simulink model "n99tot98reg50neu"  (R2022b)
settings: Solver=VariableStepAuto  StartTime=0.0  StopTime=10.0  RelTol=1e-3
libraries: neural x56
(part 2 of 2)

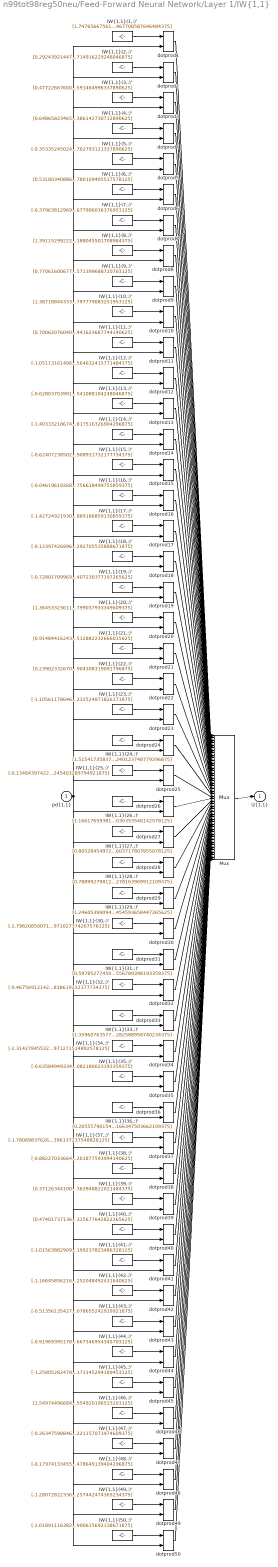
== system n99tot98reg50neu/Feed-Forward Neural Network/Layer 1/IW{1,1} ==
  "pd{1,1}" : Inport  PortDimensions=7
      mask Display: e = 0.06;c1 = [120 230 180]/255;c2 = ([120 230 180]+0)/(256+128);c3 = ([120 230 180]+128)/(256+128);patch([0 1 1 0],[0 0 1 1],c1);patch([0 1 1 1-e 1-e 0+e],[0 0 1 1-e 0+e 0+e],c2);patch([0 0 1 1-e 0+e 0+e],[0 1 1 1-e 1-e 0+e],c3);plot([0 1 1 0 0],[0 0 1 1 0]);
  "IW{1,1}(1,:)'" : Constant  Value=[1.747656675617606847339402520447038114070892333984375;0.49944644158864937022457297643995843827724456787109375;1.576232502923593070676133720553480088710784912109375;-0.265573401306849532499398947038571350276470184326171875;0.53099425991069237884545373162836767733097076416015625;-0.70547578790981491092537680742680095136165618896484375;-0.4153894187609112886860884827910922467708587646484375]
      mask Display: e = 0.06;c1 = [120 150 230]/255;c2 = ([120 150 230]+0)/383;c3 = ([120 150 230]+128)/383;patch([0 1 1 0],[0 0 1 1],c1);patch([0 1 1 1-e 1-e 0+e],[0 0 1 1-e 0+e 0+e],c2);patch([0 0 1 1-e 0+e 0+e],[0 1 1 1-e 1-e 0+e],c3);plot([0 1 1 0 0],[0 0 1 1 0]);disp('Weights');
  "IW{1,1}(10,:)'" : Constant  Value=[1.387188443330137577191862874315120279788970947265625;1.8579203813294060676497565509635023772716522216796875;-0.1472371632534580088158548960564075969159603118896484375;0.2709810301047463898527212222688831388950347900390625;-0.472918496976030555689618495307513512670993804931640625;0.277125353973486199254949724490870721638202667236328125;-0.5387110806703081511415120985475368797779083251953125]
      mask Display: e = 0.06;c1 = [120 150 230]/255;c2 = ([120 150 230]+0)/383;c3 = ([120 150 230]+128)/383;patch([0 1 1 0],[0 0 1 1],c1);patch([0 1 1 1-e 1-e 0+e],[0 0 1 1-e 0+e 0+e],c2);patch([0 0 1 1-e 0+e 0+e],[0 1 1 1-e 1-e 0+e],c3);plot([0 1 1 0 0],[0 0 1 1 0]);disp('Weights');
  "IW{1,1}(11,:)'" : Constant  Value=[0.7006207604086853724112415875424630939960479736328125;0.13393041436968455837330793656292371451854705810546875;2.002205300131398413299166350043378770351409912109375;3.592394854048140739877226224052719771862030029296875;-0.242048275446860861048747892709798179566860198974609375;-0.87313490454293984921463334103464148938655853271484375;0.79613684381734872719249551664688624441623687744140625]
      mask Display: e = 0.06;c1 = [120 150 230]/255;c2 = ([120 150 230]+0)/383;c3 = ([120 150 230]+128)/383;patch([0 1 1 0],[0 0 1 1],c1);patch([0 1 1 1-e 1-e 0+e],[0 0 1 1-e 0+e 0+e],c2);patch([0 0 1 1-e 0+e 0+e],[0 1 1 1-e 1-e 0+e],c3);plot([0 1 1 0 0],[0 0 1 1 0]);disp('Weights');
  "IW{1,1}(12,:)'" : Constant  Value=[-1.051131614068960828944909735582768917083740234375;-0.184968927308727160152557189576327800750732421875;-0.5549181350788590094680330366827547550201416015625;1.2416157312876137108759166949312202632427215576171875;-1.544207559212436020601444397470913827419281005859375;0.9759109470640339178970634748111478984355926513671875;-0.34009162520006286367646453072666190564632415771484375]
      mask Display: e = 0.06;c1 = [120 150 230]/255;c2 = ([120 150 230]+0)/383;c3 = ([120 150 230]+128)/383;patch([0 1 1 0],[0 0 1 1],c1);patch([0 1 1 1-e 1-e 0+e],[0 0 1 1-e 0+e 0+e],c2);patch([0 0 1 1-e 0+e 0+e],[0 1 1 1-e 1-e 0+e],c3);plot([0 1 1 0 0],[0 0 1 1 0]);disp('Weights');
  "IW{1,1}(13,:)'" : Constant  Value=[-0.62803703991998405253838200223981402814388275146484375;-1.8330351792178027903190695724333636462688446044921875;0.95103516127284659642526776224258355796337127685546875;-0.330923078802994929947800528680090792477130889892578125;-1.621712943876260748510276243905536830425262451171875;1.0999588154508710413637118108454160392284393310546875;0.379604016756278805910795881572994403541088104248046875]
      mask Display: e = 0.06;c1 = [120 150 230]/255;c2 = ([120 150 230]+0)/383;c3 = ([120 150 230]+128)/383;patch([0 1 1 0],[0 0 1 1],c1);patch([0 1 1 1-e 1-e 0+e],[0 0 1 1-e 0+e 0+e],c2);patch([0 0 1 1-e 0+e 0+e],[0 1 1 1-e 1-e 0+e],c3);plot([0 1 1 0 0],[0 0 1 1 0]);disp('Weights');
  "IW{1,1}(14,:)'" : Constant  Value=[-1.4033321867471306720887014307663775980472564697265625;0.28926622934015033816734785432345233857631683349609375;-0.05382639417858615937806376905427896417677402496337890625;-1.096686779105109366128090186975896358489990234375;-0.204014805347763228393631607104907743632793426513671875;0.045684822538907911282368701222367235459387302398681640625;-3.234885631069633671330620927619747817516326904296875]
      mask Display: e = 0.06;c1 = [120 150 230]/255;c2 = ([120 150 230]+0)/383;c3 = ([120 150 230]+128)/383;patch([0 1 1 0],[0 0 1 1],c1);patch([0 1 1 1-e 1-e 0+e],[0 0 1 1-e 0+e 0+e],c2);patch([0 0 1 1-e 0+e 0+e],[0 1 1 1-e 1-e 0+e],c3);plot([0 1 1 0 0],[0 0 1 1 0]);disp('Weights');
  "IW{1,1}(15,:)'" : Constant  Value=[-0.6240723850255258664532220791443251073360443115234375;0.077106870669531313300382180386804975569248199462890625;0.344852974648391763512478291886509396135807037353515625;-1.8315535668109468314668220045859925448894500732421875;1.7181195014105572482776551623828709125518798828125;1.23405048750804535728775590541772544384002685546875;1.243089227411525055089214220060966908931732177734375]
      mask Display: e = 0.06;c1 = [120 150 230]/255;c2 = ([120 150 230]+0)/383;c3 = ([120 150 230]+128)/383;patch([0 1 1 0],[0 0 1 1],c1);patch([0 1 1 1-e 1-e 0+e],[0 0 1 1-e 0+e 0+e],c2);patch([0 0 1 1-e 0+e 0+e],[0 1 1 1-e 1-e 0+e],c3);plot([0 1 1 0 0],[0 0 1 1 0]);disp('Weights');
  "IW{1,1}(16,:)'" : Constant  Value=[-0.0461961926841902015272722792360582388937473297119140625;-1.5178486125430044051398681403952650725841522216796875;0.88649917897524754817339953660848550498485565185546875;-1.694262860090099298560062379692681133747100830078125;-0.7956485499922798521055256060208193957805633544921875;-0.2040810857580830084412326641540857963263988494873046875;0.387239851931841128074296420891187153756618499755859375]
      mask Display: e = 0.06;c1 = [120 150 230]/255;c2 = ([120 150 230]+0)/383;c3 = ([120 150 230]+128)/383;patch([0 1 1 0],[0 0 1 1],c1);patch([0 1 1 1-e 1-e 0+e],[0 0 1 1-e 0+e 0+e],c2);patch([0 0 1 1-e 0+e 0+e],[0 1 1 1-e 1-e 0+e],c3);plot([0 1 1 0 0],[0 0 1 1 0]);disp('Weights');
  "IW{1,1}(17,:)'" : Constant  Value=[-1.427249219303456495566706507815979421138763427734375;0.55858969694210125478406325782998465001583099365234375;0.57312605493740698126003962897812016308307647705078125;1.6932739091869499770126594739849679172039031982421875;-0.00251143943317896738143257806541441823355853557586669921875;1.24398955198319516313176791300065815448760986328125;1.2629490962763778583166640601120889186859130859375]
      mask Display: e = 0.06;c1 = [120 150 230]/255;c2 = ([120 150 230]+0)/383;c3 = ([120 150 230]+128)/383;patch([0 1 1 0],[0 0 1 1],c1);patch([0 1 1 1-e 1-e 0+e],[0 0 1 1-e 0+e 0+e],c2);patch([0 0 1 1-e 0+e 0+e],[0 1 1 1-e 1-e 0+e],c3);plot([0 1 1 0 0],[0 0 1 1 0]);disp('Weights');
  "IW{1,1}(18,:)'" : Constant  Value=[-0.1239742699684905635759690767372376285493373870849609375;1.6475077386724310546384231201955117285251617431640625;-0.364087796388249118617608246495365165174007415771484375;1.1930065952474639967562097808695398271083831787109375;-0.7296279835965682192266967831528745591640472412109375;-1.9523779936641167953581543770269490778446197509765625;-2.11529792650099590645140779088251292705535888671875]
      mask Display: e = 0.06;c1 = [120 150 230]/255;c2 = ([120 150 230]+0)/383;c3 = ([120 150 230]+128)/383;patch([0 1 1 0],[0 0 1 1],c1);patch([0 1 1 1-e 1-e 0+e],[0 0 1 1-e 0+e 0+e],c2);patch([0 0 1 1-e 0+e 0+e],[0 1 1 1-e 1-e 0+e],c3);plot([0 1 1 0 0],[0 0 1 1 0]);disp('Weights');
  "IW{1,1}(19,:)'" : Constant  Value=[-0.72801709969798533705898080370388925075531005859375;-0.75685487829680064830739638637169264256954193115234375;-2.402055895370745819406010923557914793491363525390625;-4.40865217980332868563664305838756263256072998046875;1.788601743982917380293429232551716268062591552734375;-0.047649255890531087842543200849831919185817241668701171875;-0.54306338451648150655870495029375888407230377197265625]
      mask Display: e = 0.06;c1 = [120 150 230]/255;c2 = ([120 150 230]+0)/383;c3 = ([120 150 230]+128)/383;patch([0 1 1 0],[0 0 1 1],c1);patch([0 1 1 1-e 1-e 0+e],[0 0 1 1-e 0+e 0+e],c2);patch([0 0 1 1-e 0+e 0+e],[0 1 1 1-e 1-e 0+e],c3);plot([0 1 1 0 0],[0 0 1 1 0]);disp('Weights');
  "IW{1,1}(2,:)'" : Constant  Value=[0.2924392144750165289934784595970995724201202392578125;-1.487266421105410518777034667436964809894561767578125;1.227615355735253377389426532317884266376495361328125;0.477460046566002771495362821951857767999172210693359375;1.315340018711168124099231135915033519268035888671875;-0.493722517013425399312609442858956754207611083984375;-0.66240445347362164607574186447891406714916229248046875]
      mask Display: e = 0.06;c1 = [120 150 230]/255;c2 = ([120 150 230]+0)/383;c3 = ([120 150 230]+128)/383;patch([0 1 1 0],[0 0 1 1],c1);patch([0 1 1 1-e 1-e 0+e],[0 0 1 1-e 0+e 0+e],c2);patch([0 0 1 1-e 0+e 0+e],[0 1 1 1-e 1-e 0+e],c3);plot([0 1 1 0 0],[0 0 1 1 0]);disp('Weights');
  "IW{1,1}(20,:)'" : Constant  Value=[1.364533236116994618924991300445981323719024658203125;-1.0246759259485627158170473194331862032413482666015625;0.37029102084560083785191864080843515694141387939453125;-0.017143667388411464036490627904640859924256801605224609375;1.301862079554652940061032495577819645404815673828125;-0.73383683041816671899226776076829992234706878662109375;-0.307389929489428226361269480548799037933349609375]
      mask Display: e = 0.06;c1 = [120 150 230]/255;c2 = ([120 150 230]+0)/383;c3 = ([120 150 230]+128)/383;patch([0 1 1 0],[0 0 1 1],c1);patch([0 1 1 1-e 1-e 0+e],[0 0 1 1-e 0+e 0+e],c2);patch([0 0 1 1-e 0+e 0+e],[0 1 1 1-e 1-e 0+e],c3);plot([0 1 1 0 0],[0 0 1 1 0]);disp('Weights');
  "IW{1,1}(21,:)'" : Constant  Value=[0.9148441624371745906074693266418762505054473876953125;-2.26454895137788358994157533743418753147125244140625;0.92212391870621457368173423674306832253932952880859375;0.8388336282868242843591133350855670869350433349609375;-0.11914760626988642189250100500430562533438205718994140625;0.8434156135122823361172095246729440987110137939453125;1.3187282805795152995642638416029512882232666015625]
      mask Display: e = 0.06;c1 = [120 150 230]/255;c2 = ([120 150 230]+0)/383;c3 = ([120 150 230]+128)/383;patch([0 1 1 0],[0 0 1 1],c1);patch([0 1 1 1-e 1-e 0+e],[0 0 1 1-e 0+e 0+e],c2);patch([0 0 1 1-e 0+e 0+e],[0 1 1 1-e 1-e 0+e],c3);plot([0 1 1 0 0],[0 0 1 1 0]);disp('Weights');
  "IW{1,1}(22,:)'" : Constant  Value=[0.239023326709330297124012076892540790140628814697265625;1.63543700369563804741801504860632121562957763671875;-0.460467346974957225658187098815687932074069976806640625;-0.0152132308393917760336311317814761423505842685699462890625;1.8557407886556351872542336423066444694995880126953125;-0.145727466226683033401201328160823322832584381103515625;-1.4977839161156214498049621397512964904308319091796875]
      mask Display: e = 0.06;c1 = [120 150 230]/255;c2 = ([120 150 230]+0)/383;c3 = ([120 150 230]+128)/383;patch([0 1 1 0],[0 0 1 1],c1);patch([0 1 1 1-e 1-e 0+e],[0 0 1 1-e 0+e 0+e],c2);patch([0 0 1 1-e 0+e 0+e],[0 1 1 1-e 1-e 0+e],c3);plot([0 1 1 0 0],[0 0 1 1 0]);disp('Weights');
  "IW{1,1}(23,:)'" : Constant  Value=[-1.1056117864603602907180857073399238288402557373046875;-0.88512412117012928547410410828888416290283203125;-1.32691263005528536922383864293806254863739013671875;-0.353280134416258662088949904500623233616352081298828125;0.838270342845893967620440889731980860233306884765625;-1.1039078926360870180900519699207507073879241943359375;0.89537636960585487155839246042887680232524871826171875]
      mask Display: e = 0.06;c1 = [120 150 230]/255;c2 = ([120 150 230]+0)/383;c3 = ([120 150 230]+128)/383;patch([0 1 1 0],[0 0 1 1],c1);patch([0 1 1 1-e 1-e 0+e],[0 0 1 1-e 0+e 0+e],c2);patch([0 0 1 1-e 0+e 0+e],[0 1 1 1-e 1-e 0+e],c3);plot([0 1 1 0 0],[0 0 1 1 0]);disp('Weights');
  "IW{1,1}(24,:)'" : Constant  Value=[1.5154173583723322682459411225863732397556304931640625;1.24532548385659680434400797821581363677978515625;0.97493538415456082457666298068943433463573455810546875;-0.69399263410035072485726459490251727402210235595703125;0.28549801810493879994368171537644229829311370849609375;-0.07997892322433929057634571790913469158113002777099609375;0.64228307522436611787242100035655312240123748779296875]
      mask Display: e = 0.06;c1 = [120 150 230]/255;c2 = ([120 150 230]+0)/383;c3 = ([120 150 230]+128)/383;patch([0 1 1 0],[0 0 1 1],c1);patch([0 1 1 1-e 1-e 0+e],[0 0 1 1-e 0+e 0+e],c2);patch([0 0 1 1-e 0+e 0+e],[0 1 1 1-e 1-e 0+e],c3);plot([0 1 1 0 0],[0 0 1 1 0]);disp('Weights');
  "IW{1,1}(25,:)'" : Constant  Value=[-0.13484397422708671587798789914813823997974395751953125;-1.0885298201577475740720046815113164484500885009765625;-0.25682096877293603132130783706088550388813018798828125;0.039607047327919357726511151440718094818294048309326171875;0.11920677256356325413033658833228400908410549163818359375;-1.453256512868313254926988520310260355472564697265625;3.1420667487345621537997431005351245403289794921875]
      mask Display: e = 0.06;c1 = [120 150 230]/255;c2 = ([120 150 230]+0)/383;c3 = ([120 150 230]+128)/383;patch([0 1 1 0],[0 0 1 1],c1);patch([0 1 1 1-e 1-e 0+e],[0 0 1 1-e 0+e 0+e],c2);patch([0 0 1 1-e 0+e 0+e],[0 1 1 1-e 1-e 0+e],c3);plot([0 1 1 0 0],[0 0 1 1 0]);disp('Weights');
  "IW{1,1}(26,:)'" : Constant  Value=[1.166176593814495010548171194386668503284454345703125;1.4947985553874365560744763570255599915981292724609375;-0.54669401533347350419234089713427238166332244873046875;-2.468385339626232077847589607699774205684661865234375;0.2466663140045119162468978402102948166429996490478515625;-0.15218945163794017627623134103487245738506317138671875;-0.75219730552456021133167496373062022030353546142578125]
      mask Display: e = 0.06;c1 = [120 150 230]/255;c2 = ([120 150 230]+0)/383;c3 = ([120 150 230]+128)/383;patch([0 1 1 0],[0 0 1 1],c1);patch([0 1 1 1-e 1-e 0+e],[0 0 1 1-e 0+e 0+e],c2);patch([0 0 1 1-e 0+e 0+e],[0 1 1 1-e 1-e 0+e],c3);plot([0 1 1 0 0],[0 0 1 1 0]);disp('Weights');
  "IW{1,1}(27,:)'" : Constant  Value=[0.80528454972492713448417589461314491927623748779296875;0.58096862603202892305631621638895012438297271728515625;-1.5230858127770658949629023481975309550762176513671875;0.048101294679754651173464452540429192595183849334716796875;-1.9101916857836818142146739774034358561038970947265625;-0.294636196700321872921080057494691573083400726318359375;-1.00537860690854063960841813241131603717803955078125]
      mask Display: e = 0.06;c1 = [120 150 230]/255;c2 = ([120 150 230]+0)/383;c3 = ([120 150 230]+128)/383;patch([0 1 1 0],[0 0 1 1],c1);patch([0 1 1 1-e 1-e 0+e],[0 0 1 1-e 0+e 0+e],c2);patch([0 0 1 1-e 0+e 0+e],[0 1 1 1-e 1-e 0+e],c3);plot([0 1 1 0 0],[0 0 1 1 0]);disp('Weights');
  "IW{1,1}(28,:)'" : Constant  Value=[0.78899279812296618796807479156996123492717742919921875;-0.77936897219548451065662675318890251219272613525390625;1.6793369702174778534953247799421660602092742919921875;-0.360482007160921213984039468414266593754291534423828125;2.159602262172360287451056137797422707080841064453125;0.50602522395674631727757741828099824488162994384765625;0.74334678653509589363324039368308149278163909912109375]
      mask Display: e = 0.06;c1 = [120 150 230]/255;c2 = ([120 150 230]+0)/383;c3 = ([120 150 230]+128)/383;patch([0 1 1 0],[0 0 1 1],c1);patch([0 1 1 1-e 1-e 0+e],[0 0 1 1-e 0+e 0+e],c2);patch([0 0 1 1-e 0+e 0+e],[0 1 1 1-e 1-e 0+e],c3);plot([0 1 1 0 0],[0 0 1 1 0]);disp('Weights');
  "IW{1,1}(29,:)'" : Constant  Value=[1.246053990943079003983484653872437775135040283203125;-1.195940410100550632677141038584522902965545654296875;0.015527193852639557813954951370760682038962841033935546875;-0.01614452236154391429057142204328556545078754425048828125;1.8684337040291258968949250629520975053310394287109375;1.61290145209835866779712887364439666271209716796875;1.3569603838922239535946800970123149454593658447265625]
      mask Display: e = 0.06;c1 = [120 150 230]/255;c2 = ([120 150 230]+0)/383;c3 = ([120 150 230]+128)/383;patch([0 1 1 0],[0 0 1 1],c1);patch([0 1 1 1-e 1-e 0+e],[0 0 1 1-e 0+e 0+e],c2);patch([0 0 1 1-e 0+e 0+e],[0 1 1 1-e 1-e 0+e],c3);plot([0 1 1 0 0],[0 0 1 1 0]);disp('Weights');
  "IW{1,1}(3,:)'" : Constant  Value=[0.47722667600029800016869785395101644098758697509765625;-1.734739021348681742296093943878076970577239990234375;0.143811518424929174475579429781646467745304107666015625;1.5254287287772345660386008603381924331188201904296875;-1.094611060580545913722971818060614168643951416015625;0.400570644645104445569216977673931978642940521240234375;-0.64970032928261256532920242534601129591464996337890625]
      mask Display: e = 0.06;c1 = [120 150 230]/255;c2 = ([120 150 230]+0)/383;c3 = ([120 150 230]+128)/383;patch([0 1 1 0],[0 0 1 1],c1);patch([0 1 1 1-e 1-e 0+e],[0 0 1 1-e 0+e 0+e],c2);patch([0 0 1 1-e 0+e 0+e],[0 1 1 1-e 1-e 0+e],c3);plot([0 1 1 0 0],[0 0 1 1 0]);disp('Weights');
  "IW{1,1}(30,:)'" : Constant  Value=[-2.79820850071358773192287117126397788524627685546875;1.54179670863231788047187365009449422359466552734375;0.8064403497607031123806109462748281657695770263671875;0.351766777591807855429806295433081686496734619140625;-2.015346523677011614239518166868947446346282958984375;-1.2874435598761941879075720862601883709430694580078125;-1.4158899550481074403052161869709379971027374267578125]
      mask Display: e = 0.06;c1 = [120 150 230]/255;c2 = ([120 150 230]+0)/383;c3 = ([120 150 230]+128)/383;patch([0 1 1 0],[0 0 1 1],c1);patch([0 1 1 1-e 1-e 0+e],[0 0 1 1-e 0+e 0+e],c2);patch([0 0 1 1-e 0+e 0+e],[0 1 1 1-e 1-e 0+e],c3);plot([0 1 1 0 0],[0 0 1 1 0]);disp('Weights');
  "IW{1,1}(31,:)'" : Constant  Value=[0.59785277450840268453902126566390506923198699951171875;1.74409372320513256227059173397719860076904296875;0.354726683375673756959400861887843348085880279541015625;0.417731986711027125647177626888151280581951141357421875;-0.82909822929097909405271593641373328864574432373046875;-1.4865607481299563108478878348250873386859893798828125;-1.263156983701575253320470437756739556789398193359375]
      mask Display: e = 0.06;c1 = [120 150 230]/255;c2 = ([120 150 230]+0)/383;c3 = ([120 150 230]+128)/383;patch([0 1 1 0],[0 0 1 1],c1);patch([0 1 1 1-e 1-e 0+e],[0 0 1 1-e 0+e 0+e],c2);patch([0 0 1 1-e 0+e 0+e],[0 1 1 1-e 1-e 0+e],c3);plot([0 1 1 0 0],[0 0 1 1 0]);disp('Weights');
  "IW{1,1}(32,:)'" : Constant  Value=[-0.467569121426966216592546743413549847900867462158203125;1.071938363408374339513784434529952704906463623046875;1.1632653224053111085112277578446082770824432373046875;0.52729486405320835640253562814905308187007904052734375;1.0544362441029733190589467994868755340576171875;-0.33923970138657233430734549983753822743892669677734375;0.586796629949327464004227294935844838619232177734375]
      mask Display: e = 0.06;c1 = [120 150 230]/255;c2 = ([120 150 230]+0)/383;c3 = ([120 150 230]+128)/383;patch([0 1 1 0],[0 0 1 1],c1);patch([0 1 1 1-e 1-e 0+e],[0 0 1 1-e 0+e 0+e],c2);patch([0 0 1 1-e 0+e 0+e],[0 1 1 1-e 1-e 0+e],c3);plot([0 1 1 0 0],[0 0 1 1 0]);disp('Weights');
  "IW{1,1}(33,:)'" : Constant  Value=[1.3596076357733100081759403110481798648834228515625;-2.044468087476246864753193221986293792724609375;-1.1572914924628907584747139480896294116973876953125;-0.72656507570897621572925118016428314149379730224609375;0.42249878190688849866063492299872450530529022216796875;-1.0566425985453029579019812445039860904216766357421875;-0.82074728371824079431462450884282588958740234375]
      mask Display: e = 0.06;c1 = [120 150 230]/255;c2 = ([120 150 230]+0)/383;c3 = ([120 150 230]+128)/383;patch([0 1 1 0],[0 0 1 1],c1);patch([0 1 1 1-e 1-e 0+e],[0 0 1 1-e 0+e 0+e],c2);patch([0 0 1 1-e 0+e 0+e],[0 1 1 1-e 1-e 0+e],c3);plot([0 1 1 0 0],[0 0 1 1 0]);disp('Weights');
  "IW{1,1}(34,:)'" : Constant  Value=[-2.314278455329473072055179727612994611263275146484375;3.096416828243333529968595030368305742740631103515625;0.165424518369832906916627734972280450165271759033203125;-0.05617360352531756972904730673690210096538066864013671875;1.336202439871929659176430504885502159595489501953125;0.41390706623899287119883183549973182380199432373046875;-0.6797310280792523418114114974741823971271514892578125]
      mask Display: e = 0.06;c1 = [120 150 230]/255;c2 = ([120 150 230]+0)/383;c3 = ([120 150 230]+128)/383;patch([0 1 1 0],[0 0 1 1],c1);patch([0 1 1 1-e 1-e 0+e],[0 0 1 1-e 0+e 0+e],c2);patch([0 0 1 1-e 0+e 0+e],[0 1 1 1-e 1-e 0+e],c3);plot([0 1 1 0 0],[0 0 1 1 0]);disp('Weights');
  "IW{1,1}(35,:)'" : Constant  Value=[-0.6358494933411196203820736627676524221897125244140625;-1.5489992539573174124001297968789003789424896240234375;-1.70514848561234177992673721746541559696197509765625;-0.430721136624406308879287053059670142829418182373046875;-1.0048595441810526107673240403528325259685516357421875;-0.59747641019177766263936746327090077102184295654296875;0.43764038222769696684366635963669978082180023193359375]
      mask Display: e = 0.06;c1 = [120 150 230]/255;c2 = ([120 150 230]+0)/383;c3 = ([120 150 230]+128)/383;patch([0 1 1 0],[0 0 1 1],c1);patch([0 1 1 1-e 1-e 0+e],[0 0 1 1-e 0+e 0+e],c2);patch([0 0 1 1-e 0+e 0+e],[0 1 1 1-e 1-e 0+e],c3);plot([0 1 1 0 0],[0 0 1 1 0]);disp('Weights');
  "IW{1,1}(36,:)'" : Constant  Value=[0.205557901540687926189576728575048036873340606689453125;-1.223645094408394751184232518426142632961273193359375;0.95149708130478105605476457640179432928562164306640625;0.464250979591333601259606211897335015237331390380859375;1.3511428406536516444447215690161101520061492919921875;1.33131476326110220753662360948510468006134033203125;-1.6046192701498644961333184255636297166347503662109375]
      mask Display: e = 0.06;c1 = [120 150 230]/255;c2 = ([120 150 230]+0)/383;c3 = ([120 150 230]+128)/383;patch([0 1 1 0],[0 0 1 1],c1);patch([0 1 1 1-e 1-e 0+e],[0 0 1 1-e 0+e 0+e],c2);patch([0 0 1 1-e 0+e 0+e],[0 1 1 1-e 1-e 0+e],c3);plot([0 1 1 0 0],[0 0 1 1 0]);disp('Weights');
  "IW{1,1}(37,:)'" : Constant  Value=[-1.780898376261490057004266418516635894775390625;-0.618555182050433582929827025509439408779144287109375;-1.4373609083011322784528829288319684565067291259765625;0.90301859678045948154334610080695711076259613037109375;-0.07660094196647117270604354644092381931841373443603515625;-0.94962776800716774960875454780762083828449249267578125;0.87575113557798989205593898077495396137237548828125]
      mask Display: e = 0.06;c1 = [120 150 230]/255;c2 = ([120 150 230]+0)/383;c3 = ([120 150 230]+128)/383;patch([0 1 1 0],[0 0 1 1],c1);patch([0 1 1 1-e 1-e 0+e],[0 0 1 1-e 0+e 0+e],c2);patch([0 0 1 1-e 0+e 0+e],[0 1 1 1-e 1-e 0+e],c3);plot([0 1 1 0 0],[0 0 1 1 0]);disp('Weights');
  "IW{1,1}(38,:)'" : Constant  Value=[-0.882270336649107367321676065330393612384796142578125;0.04328286223777118302269428795625572092831134796142578125;-1.2646261397524563019345578140928409993648529052734375;0.922420917799984696472392897703684866428375244140625;-2.154867981227570172819696381338872015476226806640625;-0.966453858531078680016435100696980953216552734375;0.283468433100456496109842419173219241201877593994140625]
      mask Display: e = 0.06;c1 = [120 150 230]/255;c2 = ([120 150 230]+0)/383;c3 = ([120 150 230]+128)/383;patch([0 1 1 0],[0 0 1 1],c1);patch([0 1 1 1-e 1-e 0+e],[0 0 1 1-e 0+e 0+e],c2);patch([0 0 1 1-e 0+e 0+e],[0 1 1 1-e 1-e 0+e],c3);plot([0 1 1 0 0],[0 0 1 1 0]);disp('Weights');
  "IW{1,1}(39,:)'" : Constant  Value=[0.371263441006172756342351704006432555615901947021484375;0.53331155862665402533906444659805856645107269287109375;1.112038250172605824417360054212622344493865966796875;-0.73922509107107592374319438022212125360965728759765625;1.1841181266656504167400498772622086107730865478515625;0.9006643430544769568513174817780964076519012451171875;-1.591721705390868546459159915684722363948822021484375]
      mask Display: e = 0.06;c1 = [120 150 230]/255;c2 = ([120 150 230]+0)/383;c3 = ([120 150 230]+128)/383;patch([0 1 1 0],[0 0 1 1],c1);patch([0 1 1 1-e 1-e 0+e],[0 0 1 1-e 0+e 0+e],c2);patch([0 0 1 1-e 0+e 0+e],[0 1 1 1-e 1-e 0+e],c3);plot([0 1 1 0 0],[0 0 1 1 0]);disp('Weights');
  "IW{1,1}(4,:)'" : Constant  Value=[0.64865823465258376501196835306473076343536376953125;0.2344613740159174064547897842203383333981037139892578125;-0.48045487516191565102730010039522312581539154052734375;-1.2814031088295052551728758771787397563457489013671875;1.3399453094034914357735033263452351093292236328125;1.14153950468131082374156903824768960475921630859375;1.3336956324678974628028527149581350386142730712890625]
      mask Display: e = 0.06;c1 = [120 150 230]/255;c2 = ([120 150 230]+0)/383;c3 = ([120 150 230]+128)/383;patch([0 1 1 0],[0 0 1 1],c1);patch([0 1 1 1-e 1-e 0+e],[0 0 1 1-e 0+e 0+e],c2);patch([0 0 1 1-e 0+e 0+e],[0 1 1 1-e 1-e 0+e],c3);plot([0 1 1 0 0],[0 0 1 1 0]);disp('Weights');
  "IW{1,1}(40,:)'" : Constant  Value=[0.47401737136139654449351610310259275138378143310546875;0.1443753387717277292257023191268672235310077667236328125;-0.445205574153799521486263301994767971336841583251953125;1.4188919770855747959359405285795219242572784423828125;0.046202658139698045414167637545688194222748279571533203125;1.4128257188606887506665543696726672351360321044921875;-1.023024112720753553418262526975013315677642822265625]
      mask Display: e = 0.06;c1 = [120 150 230]/255;c2 = ([120 150 230]+0)/383;c3 = ([120 150 230]+128)/383;patch([0 1 1 0],[0 0 1 1],c1);patch([0 1 1 1-e 1-e 0+e],[0 0 1 1-e 0+e 0+e],c2);patch([0 0 1 1-e 0+e 0+e],[0 1 1 1-e 1-e 0+e],c3);plot([0 1 1 0 0],[0 0 1 1 0]);disp('Weights');
  "IW{1,1}(41,:)'" : Constant  Value=[-1.015638829099876350170461591915227472782135009765625;2.767053816463401982872483131359331309795379638671875;2.261356818364652188080299310968257486820220947265625;-0.1868634228738250413481836176288197748363018035888671875;0.719002057340242917149453205638565123081207275390625;-2.386032205980507026055192909552715718746185302734375;-5.22657363764995341881558488239534199237823486328125]
      mask Display: e = 0.06;c1 = [120 150 230]/255;c2 = ([120 150 230]+0)/383;c3 = ([120 150 230]+128)/383;patch([0 1 1 0],[0 0 1 1],c1);patch([0 1 1 1-e 1-e 0+e],[0 0 1 1-e 0+e 0+e],c2);patch([0 0 1 1-e 0+e 0+e],[0 1 1 1-e 1-e 0+e],c3);plot([0 1 1 0 0],[0 0 1 1 0]);disp('Weights');
  "IW{1,1}(42,:)'" : Constant  Value=[-1.16645856216911081304488106979988515377044677734375;-0.765914348274667755589462103671394288539886474609375;-1.147136650808885605101750115863978862762451171875;-0.4561023454182218106467416873783804476261138916015625;-1.131858827221291274867098763934336602687835693359375;-1.863473521467982951804742697277106344699859619140625;-0.48731753432313384966079183868714608252048492431640625]
      mask Display: e = 0.06;c1 = [120 150 230]/255;c2 = ([120 150 230]+0)/383;c3 = ([120 150 230]+128)/383;patch([0 1 1 0],[0 0 1 1],c1);patch([0 1 1 1-e 1-e 0+e],[0 0 1 1-e 0+e 0+e],c2);patch([0 0 1 1-e 0+e 0+e],[0 1 1 1-e 1-e 0+e],c3);plot([0 1 1 0 0],[0 0 1 1 0]);disp('Weights');
  "IW{1,1}(43,:)'" : Constant  Value=[-0.51356135427127591608353895935579203069210052490234375;-0.0380425272358840549369318750905222259461879730224609375;-1.1818972341017650595773602617555297911167144775390625;-1.6202277985747262079030406312085688114166259765625;-0.061381796748064897106811343974186456762254238128662109375;-0.12079960913816360779104996936439420096576213836669921875;1.2644207392429371861197751059080474078655242919921875]
      mask Display: e = 0.06;c1 = [120 150 230]/255;c2 = ([120 150 230]+0)/383;c3 = ([120 150 230]+128)/383;patch([0 1 1 0],[0 0 1 1],c1);patch([0 1 1 1-e 1-e 0+e],[0 0 1 1-e 0+e 0+e],c2);patch([0 0 1 1-e 0+e 0+e],[0 1 1 1-e 1-e 0+e],c3);plot([0 1 1 0 0],[0 0 1 1 0]);disp('Weights');
  "IW{1,1}(44,:)'" : Constant  Value=[-0.919693951786471064480110726435668766498565673828125;-0.63759504969468683288624788474407978355884552001953125;1.26303456644607781100830834475345909595489501953125;0.63964022040312962236185967412893660366535186767578125;0.77832391100262110494867329180124215781688690185546875;1.9202841680559898929203654915909282863140106201171875;-0.99090024817760646858033624084782786667346954345703125]
      mask Display: e = 0.06;c1 = [120 150 230]/255;c2 = ([120 150 230]+0)/383;c3 = ([120 150 230]+128)/383;patch([0 1 1 0],[0 0 1 1],c1);patch([0 1 1 1-e 1-e 0+e],[0 0 1 1-e 0+e 0+e],c2);patch([0 0 1 1-e 0+e 0+e],[0 1 1 1-e 1-e 0+e],c3);plot([0 1 1 0 0],[0 0 1 1 0]);disp('Weights');
  "IW{1,1}(45,:)'" : Constant  Value=[-1.25805282478053026551378934527747333049774169921875;0.87150745821274877567219618867966346442699432373046875;0.2542272804001601826939804595895111560821533203125;1.1438914335725669513266211652080528438091278076171875;1.5645877446592553194903985058772377669811248779296875;-0.55549203738715269285108888652757741510868072509765625;0.8576140225238664260842824660358019173145294189453125]
      mask Display: e = 0.06;c1 = [120 150 230]/255;c2 = ([120 150 230]+0)/383;c3 = ([120 150 230]+128)/383;patch([0 1 1 0],[0 0 1 1],c1);patch([0 1 1 1-e 1-e 0+e],[0 0 1 1-e 0+e 0+e],c2);patch([0 0 1 1-e 0+e 0+e],[0 1 1 1-e 1-e 0+e],c3);plot([0 1 1 0 0],[0 0 1 1 0]);disp('Weights');
  "IW{1,1}(46,:)'" : Constant  Value=[1.5497449668477685236211982555687427520751953125;-1.1408929307379047646264780269120819866657257080078125;0.35857627018847526567668637653696350753307342529296875;-2.64101483187210828162960751797072589397430419921875;1.223049071335231996471293314243666827678680419921875;1.37972539251158110573669546283781528472900390625;0.41703046322127346190455909891170449554920196533203125]
      mask Display: e = 0.06;c1 = [120 150 230]/255;c2 = ([120 150 230]+0)/383;c3 = ([120 150 230]+128)/383;patch([0 1 1 0],[0 0 1 1],c1);patch([0 1 1 1-e 1-e 0+e],[0 0 1 1-e 0+e 0+e],c2);patch([0 0 1 1-e 0+e 0+e],[0 1 1 1-e 1-e 0+e],c3);plot([0 1 1 0 0],[0 0 1 1 0]);disp('Weights');
  "IW{1,1}(47,:)'" : Constant  Value=[-0.263475988467886279575935759567073546350002288818359375;-0.86139482198021244396812790000694803893566131591796875;0.29975166291613042357511176305706612765789031982421875;1.426059500128983525968351386836729943752288818359375;0.9296813783801070041334924098919145762920379638671875;-0.46414727567939195740365221354295499622821807861328125;-0.45107432498225852324225115808076225221157073974609375]
      mask Display: e = 0.06;c1 = [120 150 230]/255;c2 = ([120 150 230]+0)/383;c3 = ([120 150 230]+128)/383;patch([0 1 1 0],[0 0 1 1],c1);patch([0 1 1 1-e 1-e 0+e],[0 0 1 1-e 0+e 0+e],c2);patch([0 0 1 1-e 0+e 0+e],[0 1 1 1-e 1-e 0+e],c3);plot([0 1 1 0 0],[0 0 1 1 0]);disp('Weights');
  "IW{1,1}(48,:)'" : Constant  Value=[-0.1797413345541949702965922597286407835781574249267578125;0.41897943081958433086953164092847146093845367431640625;-0.55505792894615446630979249675874598324298858642578125;-1.2853861057802060674504218695801682770252227783203125;-0.760985414848297292422785176313482224941253662109375;-0.951044710480042798650401891791261732578277587890625;-1.5098912287404064880291798544931225478649139404296875]
      mask Display: e = 0.06;c1 = [120 150 230]/255;c2 = ([120 150 230]+0)/383;c3 = ([120 150 230]+128)/383;patch([0 1 1 0],[0 0 1 1],c1);patch([0 1 1 1-e 1-e 0+e],[0 0 1 1-e 0+e 0+e],c2);patch([0 0 1 1-e 0+e 0+e],[0 1 1 1-e 1-e 0+e],c3);plot([0 1 1 0 0],[0 0 1 1 0]);disp('Weights');
  "IW{1,1}(49,:)'" : Constant  Value=[-1.2807282233641348323516240270691923797130584716796875;0.68915876955471688791732276513357646763324737548828125;0.2445756330386979759961008085156208835542201995849609375;1.2814935342341744473060316522605717182159423828125;0.406647322621566276179549959124415181577205657958984375;1.3771359623426366880494242650456726551055908203125;1.3778726877758324942391254808171652257442474365234375]
      mask Display: e = 0.06;c1 = [120 150 230]/255;c2 = ([120 150 230]+0)/383;c3 = ([120 150 230]+128)/383;patch([0 1 1 0],[0 0 1 1],c1);patch([0 1 1 1-e 1-e 0+e],[0 0 1 1-e 0+e 0+e],c2);patch([0 0 1 1-e 0+e 0+e],[0 1 1 1-e 1-e 0+e],c3);plot([0 1 1 0 0],[0 0 1 1 0]);disp('Weights');
  "IW{1,1}(5,:)'" : Constant  Value=[-0.353352450244067417539639563983655534684658050537109375;-0.433639085821924064045873592476709745824337005615234375;-0.90219050568865843953147987122065387666225433349609375;-0.2657325579975140517063891820725984871387481689453125;1.601768629363043761060225733672268688678741455078125;-1.3297896385042944356058569610468111932277679443359375;0.1862207972757463636526154004968702793121337890625]
      mask Display: e = 0.06;c1 = [120 150 230]/255;c2 = ([120 150 230]+0)/383;c3 = ([120 150 230]+128)/383;patch([0 1 1 0],[0 0 1 1],c1);patch([0 1 1 1-e 1-e 0+e],[0 0 1 1-e 0+e 0+e],c2);patch([0 0 1 1-e 0+e 0+e],[0 1 1 1-e 1-e 0+e],c3);plot([0 1 1 0 0],[0 0 1 1 0]);disp('Weights');
  "IW{1,1}(50,:)'" : Constant  Value=[-2.018911163828164490041672252118587493896484375;2.298443534595711046364385765627957880496978759765625;0.33520956691234216062724726725718937814235687255859375;1.2034240760566057293345920697902329266071319580078125;1.5925325800665455222571154081379063427448272705078125;-0.3031269859191016990962452837266027927398681640625;0.373687957622833522020044938471983186900615692138671875]
      mask Display: e = 0.06;c1 = [120 150 230]/255;c2 = ([120 150 230]+0)/383;c3 = ([120 150 230]+128)/383;patch([0 1 1 0],[0 0 1 1],c1);patch([0 1 1 1-e 1-e 0+e],[0 0 1 1-e 0+e 0+e],c2);patch([0 0 1 1-e 0+e 0+e],[0 1 1 1-e 1-e 0+e],c3);plot([0 1 1 0 0],[0 0 1 1 0]);disp('Weights');
  "IW{1,1}(6,:)'" : Constant  Value=[0.5318034088629299827033491965266875922679901123046875;-0.05717590530931339343201358360602171160280704498291015625;-0.94733840130549895608425003956654109060764312744140625;-0.0146788195354180840690450082774987095035612583160400390625;2.308522830923596114161000514286570250988006591796875;1.2037431893397132487422140911803580820560455322265625;-0.03790454788108706118965329778802697546780109405517578125]
      mask Display: e = 0.06;c1 = [120 150 230]/255;c2 = ([120 150 230]+0)/383;c3 = ([120 150 230]+128)/383;patch([0 1 1 0],[0 0 1 1],c1);patch([0 1 1 1-e 1-e 0+e],[0 0 1 1-e 0+e 0+e],c2);patch([0 0 1 1-e 0+e 0+e],[0 1 1 1-e 1-e 0+e],c3);plot([0 1 1 0 0],[0 0 1 1 0]);disp('Weights');
  "IW{1,1}(7,:)'" : Constant  Value=[-0.379638129699689186313804611927480436861515045166015625;0.5398169246130877230172018244047649204730987548828125;1.140584439302090746792828213074244558811187744140625;0.61722127131611637107511114663793705403804779052734375;1.3606223929806964267896773890242911875247955322265625;0.56343294578792069149386634308029897511005401611328125;0.97896543814351677514906668875482864677906036376953125]
      mask Display: e = 0.06;c1 = [120 150 230]/255;c2 = ([120 150 230]+0)/383;c3 = ([120 150 230]+128)/383;patch([0 1 1 0],[0 0 1 1],c1);patch([0 1 1 1-e 1-e 0+e],[0 0 1 1-e 0+e 0+e],c2);patch([0 0 1 1-e 0+e 0+e],[0 1 1 1-e 1-e 0+e],c3);plot([0 1 1 0 0],[0 0 1 1 0]);disp('Weights');
  "IW{1,1}(8,:)'" : Constant  Value=[1.3911529922247594104334211806417442858219146728515625;-3.108901065696418442030335427261888980865478515625;-2.56068493120445506150417713797651231288909912109375;-0.476377804219743572478051873986260034143924713134765625;0.5930594051890292206508092931471765041351318359375;-1.5123935503399625890352808710304088890552520751953125;0.958351638789282755936937974183820188045501708984375]
      mask Display: e = 0.06;c1 = [120 150 230]/255;c2 = ([120 150 230]+0)/383;c3 = ([120 150 230]+128)/383;patch([0 1 1 0],[0 0 1 1],c1);patch([0 1 1 1-e 1-e 0+e],[0 0 1 1-e 0+e 0+e],c2);patch([0 0 1 1-e 0+e 0+e],[0 1 1 1-e 1-e 0+e],c3);plot([0 1 1 0 0],[0 0 1 1 0]);disp('Weights');
  "IW{1,1}(9,:)'" : Constant  Value=[0.770616006774930806244583436637185513973236083984375;-1.3223955779284024547592935050488449633121490478515625;-1.6183259513531871309766074773506261408329010009765625;1.5763537694544391687401230228715576231479644775390625;-1.1200073332976734352683934048400260508060455322265625;1.4510169135761297187769969241344369947910308837890625;0.7298236116551006791297595555079169571399688720703125]
      mask Display: e = 0.06;c1 = [120 150 230]/255;c2 = ([120 150 230]+0)/383;c3 = ([120 150 230]+128)/383;patch([0 1 1 0],[0 0 1 1],c1);patch([0 1 1 1-e 1-e 0+e],[0 0 1 1-e 0+e 0+e],c2);patch([0 0 1 1-e 0+e 0+e],[0 1 1 1-e 1-e 0+e],c3);plot([0 1 1 0 0],[0 0 1 1 0]);disp('Weights');
  Mux : Mux  Inputs=50
      mask Display: e = 0.06;c1 = [120 150 230]/255;c2 = ([120 150 230]+0)/383;c3 = ([120 150 230]+128)/383;patch([0 1 1 0],[0 0 1 1],c1);patch([0 1 1 1-e 1-e 0+e],[0 0 1 1-e 0+e 0+e],c2);patch([0 0 1 1-e 0+e 0+e],[0 1 1 1-e 1-e 0+e],c3);plot([0 1 1 0 0],[0 0 1 1 0]);disp('Mux');
  dotprod{1..50} (50 alike) : neural/Weight Functions/dotprod
  "iz{1,1}" : Outport
      mask Display: e = 0.06;c1 = [120 230 180]/255;c2 = ([120 230 180]+0)/(256+128);c3 = ([120 230 180]+128)/(256+128);patch([0 1 1 0],[0 0 1 1],c1);patch([0 1 1 1-e 1-e 0+e],[0 0 1 1-e 0+e 0+e],c2);patch([0 0 1 1-e 0+e 0+e],[0 1 1 1-e 1-e 0+e],c3);plot([0 1 1 0 0],[0 0 1 1 0]);
  wires:
  "IW{1,1}(1,:)'"/1 -> dotprod1/1
  "pd{1,1}"/1 -> dotprod1/2, dotprod2/2, dotprod3/2, dotprod4/2, dotprod5/2, dotprod6/2, dotprod7/2, dotprod8/2, dotprod9/2, dotprod10/2, dotprod11/2, dotprod12/2, dotprod13/2, dotprod14/2, dotprod15/2, dotprod16/2, dotprod17/2, dotprod18/2, dotprod19/2, dotprod20/2, dotprod21/2, dotprod22/2, dotprod23/2, dotprod24/2, dotprod25/2, dotprod26/2, dotprod27/2, dotprod28/2, dotprod29/2, dotprod30/2, dotprod31/2, dotprod32/2, dotprod33/2, dotprod34/2, dotprod35/2, dotprod36/2, dotprod37/2, dotprod38/2, dotprod39/2, dotprod40/2, dotprod41/2, dotprod42/2, dotprod43/2, dotprod44/2, dotprod45/2, dotprod46/2, dotprod47/2, dotprod48/2, dotprod49/2, dotprod50/2
  dotprod1/1 -> Mux/1
  "IW{1,1}(2,:)'"/1 -> dotprod2/1
  dotprod2/1 -> Mux/2
  "IW{1,1}(3,:)'"/1 -> dotprod3/1
  dotprod3/1 -> Mux/3
  "IW{1,1}(4,:)'"/1 -> dotprod4/1
  dotprod4/1 -> Mux/4
  "IW{1,1}(5,:)'"/1 -> dotprod5/1
  dotprod5/1 -> Mux/5
  "IW{1,1}(6,:)'"/1 -> dotprod6/1
  dotprod6/1 -> Mux/6
  "IW{1,1}(7,:)'"/1 -> dotprod7/1
  dotprod7/1 -> Mux/7
  "IW{1,1}(8,:)'"/1 -> dotprod8/1
  dotprod8/1 -> Mux/8
  "IW{1,1}(9,:)'"/1 -> dotprod9/1
  dotprod9/1 -> Mux/9
  "IW{1,1}(10,:)'"/1 -> dotprod10/1
  dotprod10/1 -> Mux/10
  "IW{1,1}(11,:)'"/1 -> dotprod11/1
  dotprod11/1 -> Mux/11
  "IW{1,1}(12,:)'"/1 -> dotprod12/1
  dotprod12/1 -> Mux/12
  "IW{1,1}(13,:)'"/1 -> dotprod13/1
  dotprod13/1 -> Mux/13
  "IW{1,1}(14,:)'"/1 -> dotprod14/1
  dotprod14/1 -> Mux/14
  "IW{1,1}(15,:)'"/1 -> dotprod15/1
  dotprod15/1 -> Mux/15
  "IW{1,1}(16,:)'"/1 -> dotprod16/1
  dotprod16/1 -> Mux/16
  "IW{1,1}(17,:)'"/1 -> dotprod17/1
  dotprod17/1 -> Mux/17
  "IW{1,1}(18,:)'"/1 -> dotprod18/1
  dotprod18/1 -> Mux/18
  "IW{1,1}(19,:)'"/1 -> dotprod19/1
  dotprod19/1 -> Mux/19
  "IW{1,1}(20,:)'"/1 -> dotprod20/1
  dotprod20/1 -> Mux/20
  "IW{1,1}(21,:)'"/1 -> dotprod21/1
  dotprod21/1 -> Mux/21
  "IW{1,1}(22,:)'"/1 -> dotprod22/1
  dotprod22/1 -> Mux/22
  "IW{1,1}(23,:)'"/1 -> dotprod23/1
  dotprod23/1 -> Mux/23
  "IW{1,1}(24,:)'"/1 -> dotprod24/1
  dotprod24/1 -> Mux/24
  "IW{1,1}(25,:)'"/1 -> dotprod25/1
  dotprod25/1 -> Mux/25
  "IW{1,1}(26,:)'"/1 -> dotprod26/1
  dotprod26/1 -> Mux/26
  "IW{1,1}(27,:)'"/1 -> dotprod27/1
  dotprod27/1 -> Mux/27
  "IW{1,1}(28,:)'"/1 -> dotprod28/1
  dotprod28/1 -> Mux/28
  "IW{1,1}(29,:)'"/1 -> dotprod29/1
  dotprod29/1 -> Mux/29
  "IW{1,1}(30,:)'"/1 -> dotprod30/1
  dotprod30/1 -> Mux/30
  "IW{1,1}(31,:)'"/1 -> dotprod31/1
  dotprod31/1 -> Mux/31
  "IW{1,1}(32,:)'"/1 -> dotprod32/1
  dotprod32/1 -> Mux/32
  "IW{1,1}(33,:)'"/1 -> dotprod33/1
  dotprod33/1 -> Mux/33
  "IW{1,1}(34,:)'"/1 -> dotprod34/1
  dotprod34/1 -> Mux/34
  "IW{1,1}(35,:)'"/1 -> dotprod35/1
  dotprod35/1 -> Mux/35
  "IW{1,1}(36,:)'"/1 -> dotprod36/1
  dotprod36/1 -> Mux/36
  "IW{1,1}(37,:)'"/1 -> dotprod37/1
  dotprod37/1 -> Mux/37
  "IW{1,1}(38,:)'"/1 -> dotprod38/1
  dotprod38/1 -> Mux/38
  "IW{1,1}(39,:)'"/1 -> dotprod39/1
  dotprod39/1 -> Mux/39
  "IW{1,1}(40,:)'"/1 -> dotprod40/1
  dotprod40/1 -> Mux/40
  "IW{1,1}(41,:)'"/1 -> dotprod41/1
  dotprod41/1 -> Mux/41
  "IW{1,1}(42,:)'"/1 -> dotprod42/1
  dotprod42/1 -> Mux/42
  "IW{1,1}(43,:)'"/1 -> dotprod43/1
  dotprod43/1 -> Mux/43
  "IW{1,1}(44,:)'"/1 -> dotprod44/1
  dotprod44/1 -> Mux/44
  "IW{1,1}(45,:)'"/1 -> dotprod45/1
  dotprod45/1 -> Mux/45
  "IW{1,1}(46,:)'"/1 -> dotprod46/1
  dotprod46/1 -> Mux/46
  "IW{1,1}(47,:)'"/1 -> dotprod47/1
  dotprod47/1 -> Mux/47
  "IW{1,1}(48,:)'"/1 -> dotprod48/1
  dotprod48/1 -> Mux/48
  "IW{1,1}(49,:)'"/1 -> dotprod49/1
  dotprod49/1 -> Mux/49
  "IW{1,1}(50,:)'"/1 -> dotprod50/1
  dotprod50/1 -> Mux/50
  Mux/1 -> "iz{1,1}"/1

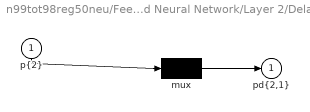
== system n99tot98reg50neu/Feed-Forward Neural Network/Layer 2/Delays 1 ==
  "p{2}" : Inport  PortDimensions=50
      mask Display: e = 0.06;c1 = [120 230 180]/255;c2 = ([120 230 180]+0)/(256+128);c3 = ([120 230 180]+128)/(256+128);patch([0 1 1 0],[0 0 1 1],c1);patch([0 1 1 1-e 1-e 0+e],[0 0 1 1-e 0+e 0+e],c2);patch([0 0 1 1-e 0+e 0+e],[0 1 1 1-e 1-e 0+e],c3);plot([0 1 1 0 0],[0 0 1 1 0]);
  mux : Mux  Inputs=1
      mask Display: e = 0.06;c1 = [120 150 230]/255;c2 = ([120 150 230]+0)/383;c3 = ([120 150 230]+128)/383;patch([0 1 1 0],[0 0 1 1],c1);patch([0 1 1 1-e 1-e 0+e],[0 0 1 1-e 0+e 0+e],c2);patch([0 0 1 1-e 0+e 0+e],[0 1 1 1-e 1-e 0+e],c3);plot([0 1 1 0 0],[0 0 1 1 0]);disp('Mux')
  "pd{2,1}" : Outport
      mask Display: e = 0.06;c1 = [120 230 180]/255;c2 = ([120 230 180]+0)/(256+128);c3 = ([120 230 180]+128)/(256+128);patch([0 1 1 0],[0 0 1 1],c1);patch([0 1 1 1-e 1-e 0+e],[0 0 1 1-e 0+e 0+e],c2);patch([0 0 1 1-e 0+e 0+e],[0 1 1 1-e 1-e 0+e],c3);plot([0 1 1 0 0],[0 0 1 1 0]);
  wires:
  "p{2}"/1 -> mux/1
  mux/1 -> "pd{2,1}"/1

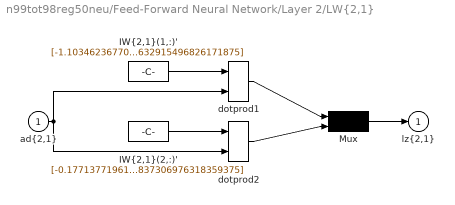
== system n99tot98reg50neu/Feed-Forward Neural Network/Layer 2/LW{2,1} ==
  "ad{2,1}" : Inport  PortDimensions=50
      mask Display: e = 0.06;c1 = [120 230 180]/255;c2 = ([120 230 180]+0)/(256+128);c3 = ([120 230 180]+128)/(256+128);patch([0 1 1 0],[0 0 1 1],c1);patch([0 1 1 1-e 1-e 0+e],[0 0 1 1-e 0+e 0+e],c2);patch([0 0 1 1-e 0+e 0+e],[0 1 1 1-e 1-e 0+e],c3);plot([0 1 1 0 0],[0 0 1 1 0]);
  "IW{2,1}(1,:)'" : Constant  Value=[-1.103462367703454294343146102619357407093048095703125;-0.173389462198645871726654377198428846895694732666015625;0.64683998304327838813065909562283195555210113525390625;1.151073103183495760504229110665619373321533203125;-0.411704790475478088485061789469909854233264923095703125;-1.4187693531356744269800174151896499097347259521484375;-0.40842696138575973474615921077202074229717254638671875;0.98291123342178376987021692912094295024871826171875;-0.940678257214297541821679260465316474437713623046875;-0.00010816373542705203479596942628404576680622994899749755859375;2.050360643931851800658705542446114122867584228515625;-0.99225815139485684657216779669397510588169097900390625;-1.1791208066892331363106904973392374813556671142578125;-0.90422040946100457059486643629497848451137542724609375;0.60922192362671889753755749552510678768157958984375;-0.280182588620675243618052263627760112285614013671875;1.0670100736571175303879499551840126514434814453125;1.0273148801777092220532949795597232878208160400390625;3.37315181240567785181383442250080406665802001953125;-1.387161215388457602415428482345305383205413818359375;1.6852468263890976185592762703890912234783172607421875;0.62632842992243187296708128997124731540679931640625;-0.407997151136406277505130901772645302116870880126953125;-0.94616588400781564960340119796455837786197662353515625;-1.27438810537446034487629731302149593830108642578125;0.7589541631164860024938434435171075165271759033203125;-0.8598655230186069697850825832574628293514251708984375;-1.103732928383181377540722678531892597675323486328125;-1.6459161376534925391723618304240517318248748779296875;-1.651715828856747947384064900688827037811279296875;0.478620948935355061681917732130386866629123687744140625;0.2723637562500258457731661110301502048969268798828125;0.9371937651799502333460623049177229404449462890625;1.2916748837337783673007152174250222742557525634765625;0.49684247192367869683238268407876603305339813232421875;1.07638572501492735256078958627767860889434814453125;-0.7646662195951414719985450574313290417194366455078125;-0.48960405943661211569661872999859042465686798095703125;-0.346370179660698218615522137042717076838016510009765625;0.2459578415226557346340285903352196328341960906982421875;-1.414777225172336283520735378260724246501922607421875;1.0981868436513797515630130874342285096645355224609375;0.88650488763662405045096193134668283164501190185546875;1.32846766168543783948052805499173700809478759765625;1.5810299167087695781930278826621361076831817626953125;1.4585933638880523854908233261085115373134613037109375;-0.68748072050419839484902695403434336185455322265625;-0.5731175710696108094310829983442090451717376708984375;0.843276631759791062137310291291214525699615478515625;-1.182860125915009774644204298965632915496826171875]
      mask Display: e = 0.06;c1 = [120 150 230]/255;c2 = ([120 150 230]+0)/383;c3 = ([120 150 230]+128)/383;patch([0 1 1 0],[0 0 1 1],c1);patch([0 1 1 1-e 1-e 0+e],[0 0 1 1-e 0+e 0+e],c2);patch([0 0 1 1-e 0+e 0+e],[0 1 1 1-e 1-e 0+e],c3);plot([0 1 1 0 0],[0 0 1 1 0]);disp('weights');
  "IW{2,1}(2,:)'" : Constant  Value=[-0.1771377196183677449337068310342147015035152435302734375;-0.04969687446930164120839634733783896081149578094482421875;0.90663431826319762496524390371632762253284454345703125;0.0939291387847450975900898129111737944185733795166015625;-0.70383401522498345581624334954540245234966278076171875;0.389695659529671944998341359678306616842746734619140625;0.31129345920001671998988967970944941043853759765625;-0.263428397644382139564100953066372312605381011962890625;0.075821568827941998591768424375914037227630615234375;-0.80611865736607890564613398964866064488887786865234375;0.334314342080233195542149360335315577685832977294921875;0.1126995363301433183966793194485944695770740509033203125;0.425293754905475385186264247749932110309600830078125;-0.280392496353138509501690123215666972100734710693359375;0.1872126032276421880862216085006366483867168426513671875;-0.646412130765089187889316235668957233428955078125;-0.5426251273292559407224189271801151335239410400390625;-0.164099991364381636582692181036691181361675262451171875;0.1945288183541095394790687578279175795614719390869140625;-0.60971326335464615109316355301416479051113128662109375;-0.375292854068967340896989526299876160919666290283203125;-0.7300155530356386979207172771566547453403472900390625;0.425625785850662186060588965119677595794200897216796875;-0.25148923085304131230799384866259060800075531005859375;0.1418534571470476957077977431254112161695957183837890625;0.73529394258056790523170320739154703915119171142578125;-1.0853350186014580902593706923653371632099151611328125;-0.6506057657172288344327171216718852519989013671875;0.30492484754041537797775163198821246623992919921875;0.1334112749210038806335631988986278884112834930419921875;1.259042873201923651294009687262587249279022216796875;-0.344455499814267318559046771042631007730960845947265625;0.418728820897241560405888094464899040758609771728515625;-0.488482605260070756880708131575374864041805267333984375;0.030244348221037553603451897288323380053043365478515625;0.0091600155503559384240208629535118234343826770782470703125;-0.5121598245255636339123839206877164542675018310546875;-0.904908741395510585192596408887766301631927490234375;-0.467759130337242978736611576096038334071636199951171875;-0.3919660314734423334215307477279566228389739990234375;-0.280109786604913535423833081949851475656032562255859375;0.002757485074899639933276862535649343044497072696685791015625;0.207678618929289182659658763441257178783416748046875;0.41948485462201390294723069018800742924213409423828125;0.0061474724868368253727357597426816937513649463653564453125;-0.397867692579844611788786323813837952911853790283203125;-0.357085252563309418771808623205288313329219818115234375;-0.49501292581586742169719173034536652266979217529296875;-0.72477627963568636015878610123763792216777801513671875;0.8136465460232213953162272446206770837306976318359375]
      mask Display: e = 0.06;c1 = [120 150 230]/255;c2 = ([120 150 230]+0)/383;c3 = ([120 150 230]+128)/383;patch([0 1 1 0],[0 0 1 1],c1);patch([0 1 1 1-e 1-e 0+e],[0 0 1 1-e 0+e 0+e],c2);patch([0 0 1 1-e 0+e 0+e],[0 1 1 1-e 1-e 0+e],c3);plot([0 1 1 0 0],[0 0 1 1 0]);disp('weights');
  Mux : Mux  Inputs=2
      mask Display: e = 0.06;c1 = [120 150 230]/255;c2 = ([120 150 230]+0)/383;c3 = ([120 150 230]+128)/383;patch([0 1 1 0],[0 0 1 1],c1);patch([0 1 1 1-e 1-e 0+e],[0 0 1 1-e 0+e 0+e],c2);patch([0 0 1 1-e 0+e 0+e],[0 1 1 1-e 1-e 0+e],c3);plot([0 1 1 0 0],[0 0 1 1 0]);disp('Mux');
  dotprod1 : neural/Weight Functions/dotprod
  dotprod2 : neural/Weight Functions/dotprod
  "lz{2,1}" : Outport
      mask Display: e = 0.06;c1 = [120 230 180]/255;c2 = ([120 230 180]+0)/(256+128);c3 = ([120 230 180]+128)/(256+128);patch([0 1 1 0],[0 0 1 1],c1);patch([0 1 1 1-e 1-e 0+e],[0 0 1 1-e 0+e 0+e],c2);patch([0 0 1 1-e 0+e 0+e],[0 1 1 1-e 1-e 0+e],c3);plot([0 1 1 0 0],[0 0 1 1 0]);
  wires:
  "IW{2,1}(1,:)'"/1 -> dotprod1/1
  "ad{2,1}"/1 -> dotprod1/2, dotprod2/2
  dotprod1/1 -> Mux/1
  "IW{2,1}(2,:)'"/1 -> dotprod2/1
  dotprod2/1 -> Mux/2
  Mux/1 -> "lz{2,1}"/1
